simulink model "pmsw_modeling"  (R2023a)
settings: Solver=FixedStepAuto  StartTime=0.0  StopTime=10.0  FixedStep=1e-3  RelTol=1e-3
libraries: simulink x1
settings Model: Creator=ItShop  LastModifiedBy=ItShop

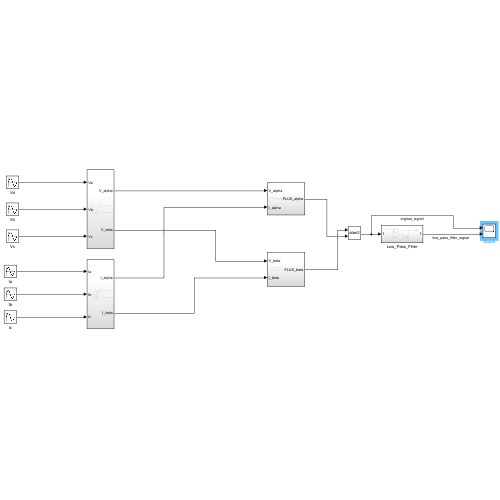
[thumbnail: Simulink's stored preview of the top-level diagram]
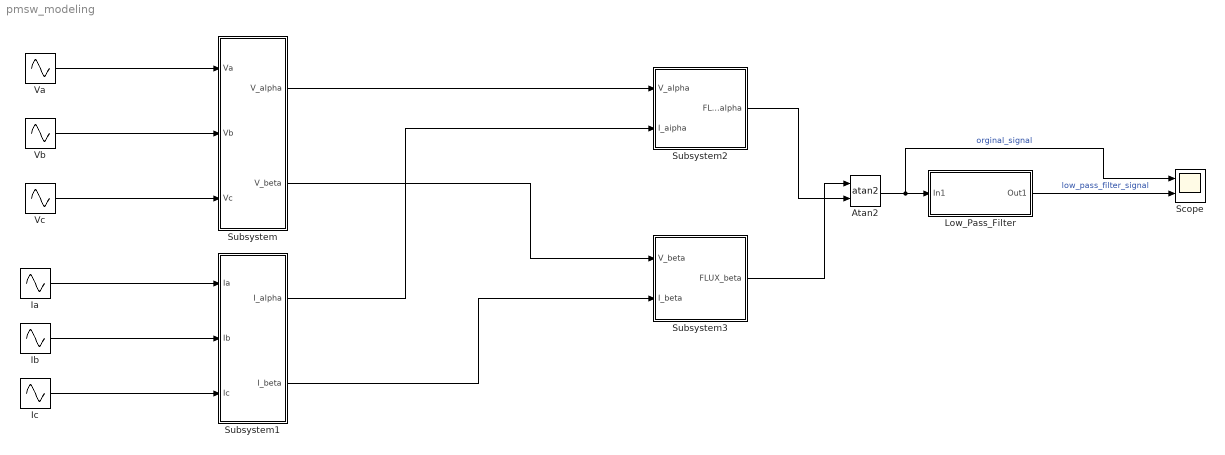
== system pmsw_modeling ==
  Atan2 : Trigonometry  Operator=atan2
  Ia : Sin  Amplitude=2  Frequency=300  SampleTime=0
  Ib : Sin  Amplitude=2  Frequency=300  Phase=-120*(pi/180)  SampleTime=0
  Ic : Sin  Amplitude=2  Frequency=300  Phase=120*(pi/180)  SampleTime=0
  Low_Pass_Filter : Subsystem
  Scope : Scope  NumInputPorts=2
  Subsystem : Subsystem
  Subsystem1 : Subsystem
  Subsystem2 : Subsystem
  Subsystem3 : Subsystem
  Va : Sin  Amplitude=12  Frequency=300  SampleTime=0
  Vb : Sin  Amplitude=12  Frequency=300  Phase=-120*(pi/180)  SampleTime=0
  Vc : Sin  Amplitude=12  Frequency=300  Phase=120*(pi/180)  SampleTime=0
  wires:
  Va/1 -> Subsystem/1(Va)
  Vb/1 -> Subsystem/2(Vb)
  Vc/1 -> Subsystem/3(Vc)
  Ia/1 -> Subsystem1/1(Ia)
  Ib/1 -> Subsystem1/2(Ib)
  Ic/1 -> Subsystem1/3(Ic)
  Subsystem/1(V_alpha) -> Subsystem2/1(V_alpha)
  Subsystem1/1(I_alpha) -> Subsystem2/2(I_aipha)
  Subsystem/2(V_beta) -> Subsystem3/1(V_beta)
  Subsystem1/2(I_beta) -> Subsystem3/2(I_beta)
  Subsystem2/1(FLUX_alpha) -> Atan2/2
  Subsystem3/1(FLUX_beta) -> Atan2/1
  Atan2/1 -> Scope/1, Low_Pass_Filter/1(In1)  "orginal_signal"
  Low_Pass_Filter/1(Out1) -> Scope/2  "low_pass_filter_signal"

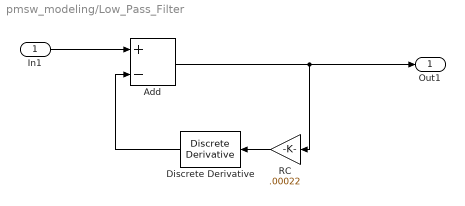
== system pmsw_modeling/Low_Pass_Filter ==
  In1 : Inport
  Add : Sum  Inputs=+-
  Discrete Derivative : simulink/Discrete/Discrete Derivative  gainval=1.0  ICPrevScaledInput=0.0  OutMin=[]  OutMax=[]  OutDataType=fixdt(1, 16)  OutScaling=2^-10  DoSatur=off
  RC : Gain  Gain=.00022
  Out1 : Outport
  wires:
  In1/1 -> Add/1
  Add/1 -> RC/1, Out1/1
  Discrete Derivative/1 -> Add/2
  RC/1 -> Discrete Derivative/1

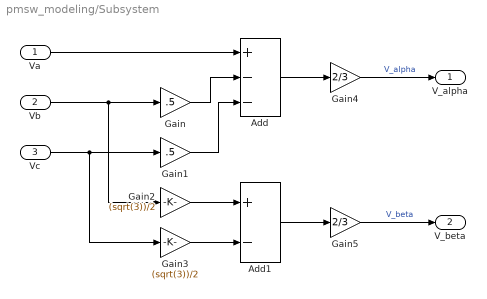
== system pmsw_modeling/Subsystem ==
  Va : Inport
  Vb : Inport  Port=2
  Vc : Inport  Port=3
  Add : Sum  Inputs=+--
  Add1 : Sum  Inputs=+-
  Gain : Gain  Gain=.5
  Gain1 : Gain  Gain=.5
  Gain2 : Gain  Gain=(sqrt(3))/2
  Gain3 : Gain  Gain=(sqrt(3))/2
  Gain4 : Gain  Gain=2/3
  Gain5 : Gain  Gain=2/3
  V_alpha : Outport
  V_beta : Outport  Port=2
  wires:
  Vb/1 -> Gain2/1, Gain/1
  Add1/1 -> Gain5/1
  Vc/1 -> Gain3/1, Gain1/1
  Add/1 -> Gain4/1
  Gain2/1 -> Add1/1
  Gain3/1 -> Add1/2
  Gain/1 -> Add/2
  Gain1/1 -> Add/3
  Gain5/1 -> V_beta/1  "V_beta"
  Va/1 -> Add/1
  Gain4/1 -> V_alpha/1  "V_alpha"

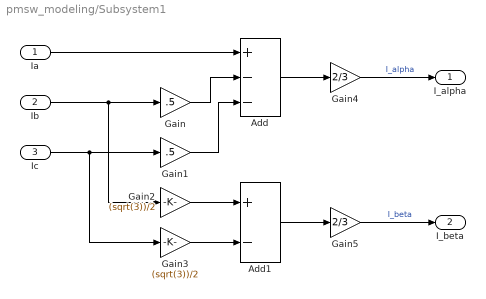
== system pmsw_modeling/Subsystem1 ==
  Ia : Inport
  Ib : Inport  Port=2
  Ic : Inport  Port=3
  Add : Sum  Inputs=+--
  Add1 : Sum  Inputs=+-
  Gain : Gain  Gain=.5
  Gain1 : Gain  Gain=.5
  Gain2 : Gain  Gain=(sqrt(3))/2
  Gain3 : Gain  Gain=(sqrt(3))/2
  Gain4 : Gain  Gain=2/3
  Gain5 : Gain  Gain=2/3
  I_alpha : Outport
  I_beta : Outport  Port=2
  wires:
  Gain4/1 -> I_alpha/1  "I_alpha"
  Ia/1 -> Add/1
  Gain5/1 -> I_beta/1  "I_beta"
  Gain1/1 -> Add/3
  Gain/1 -> Add/2
  Gain3/1 -> Add1/2
  Gain2/1 -> Add1/1
  Add/1 -> Gain4/1
  Ic/1 -> Gain1/1, Gain3/1
  Add1/1 -> Gain5/1
  Ib/1 -> Gain/1, Gain2/1

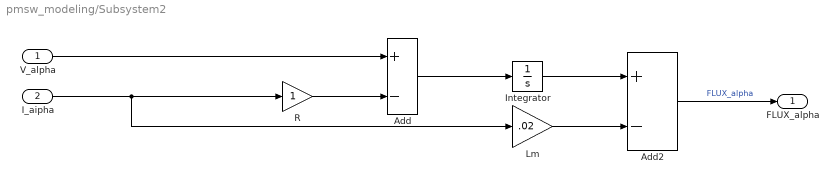
== system pmsw_modeling/Subsystem2 ==
  V_alpha : Inport
  I_aipha : Inport  Port=2
  Add : Sum  Inputs=+-
  Add2 : Sum  Inputs=+-
  Integrator : Integrator
  Lm : Gain  Gain=.02
  R : Gain
  FLUX_alpha : Outport
  wires:
  Integrator/1 -> Add2/1
  I_aipha/1 -> Lm/1, R/1
  R/1 -> Add/2
  Lm/1 -> Add2/2
  Add2/1 -> FLUX_alpha/1  "FLUX_alpha"
  Add/1 -> Integrator/1
  V_alpha/1 -> Add/1

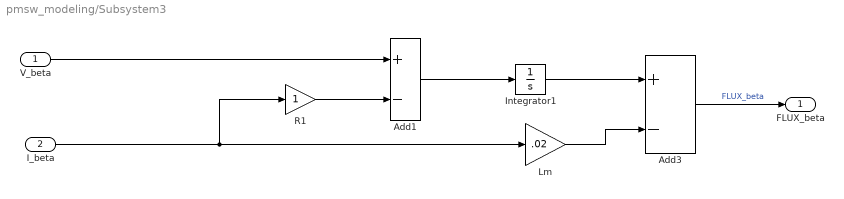
== system pmsw_modeling/Subsystem3 ==
  V_beta : Inport
  I_beta : Inport  Port=2
  Add1 : Sum  Inputs=+-
  Add3 : Sum  Inputs=+-
  Integrator1 : Integrator
  Lm : Gain  Gain=.02
  R1 : Gain
  FLUX_beta : Outport
  wires:
  V_beta/1 -> Add1/1
  Lm/1 -> Add3/2
  R1/1 -> Add1/2
  I_beta/1 -> Lm/1, R1/1
  Integrator1/1 -> Add3/1
  Add1/1 -> Integrator1/1
  Add3/1 -> FLUX_beta/1  "FLUX_beta"
